simulink model "simu_rst_pendule"  (R2025b)
settings: Solver=ode45  StartTime=0.0  StopTime=30  MaxStep=0.01  RelTol=1e-3  EnableMultiTasking=on
undefined symbols (not defined in the file): g, H, l, R, S, sigbuilder_block, T
settings Model: Creator=2022-0702  LastModifiedBy=baki
settings SolverCC: AlgebraicLoopSolver=TrustRegion
settings DataIOCC: LimitDataPoints=on  SaveFormat=Array  SignalLoggingSaveFormat=ModelDataLogs  ReturnWorkspaceOutputs=off
settings OptimizationCC: InitFltsAndDblsToZero=on  LifeSpan=inf
settings DebuggingCC: SaveWithParameterizedLinksMsg=none  UnderspecifiedInitializationDetection=Classic  MergeDetectMultiDrivingBlocksExec=none  SignalResolutionControl=TryResolveAllWithWarning  SolverPrmCheckMsg=warning  MultiTaskDSMMsg=warning  MultiTaskCondExecSysMsg=none  FcnCallInpInsideContextMsg=warning  UnconnectedInputMsg=warning  UnconnectedOutputMsg=warning  UnconnectedLineMsg=warning  SFUnexpectedBacktrackingDiag=warning  SFNoUnconditionalDefaultTransitionDiag=warning  SFExecutionAtInitializationDiag=none  ArithmeticOperatorsInVariantConditions=warning
settings HardwareCC: ProdBitPerPointer=32.0  ProdBitPerSizeT=32.0  ProdBitPerPtrDiffT=32.0  ProdLargestAtomicFloat=None  ProdIntDivRoundTo=Undefined  ProdEndianess=Unspecified  ProdWordSize=32.0  ProdHWDeviceType=32-bit Generic
settings ModelReferenceCC: PropagateSignalLabelsOutOfModel=off
settings SFSimCC: SimUseLocalCustomCode=off  CustomCodeUndefinedFunction=UseInterfaceOnly
settings RTWCC: RTWUseLocalCustomCode=off  GPUComputeCapability=3.5
settings CodeAppCC: StateflowObjectComments=on
settings GRTTargetCC: TargetFcnLib=ansi_tfl_tmw.mat  TargetLangStandard=C89/C90 (ANSI)  CombineOutputUpdateFcns=off  GRTInterface=on
settings ConfigComp: CovMetricSettings=dw  CovSaveCumulativeToWorkspaceVar=on  CovSaveSingleToWorkspaceVar=on  CovExternalEMLEnable=off

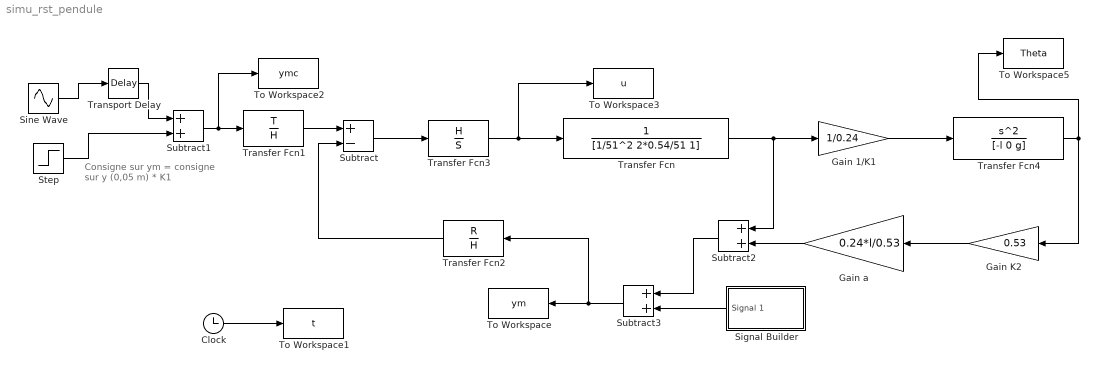
== system simu_rst_pendule ==
  note: Consigne sur ym
      | = consigne sur y
      | (0,05 m) * K1
  Clock : Clock
  Gain 1/K1 : Gain  Gain=1/0.24
  Gain K2 : Gain  Gain=0.53
  Gain a : Gain  Gain=0.24*l/0.53
  Signal Builder : Subsystem  Tag=STV Subsys  LoadFcn=sigbuilder_block('load');  StartFcn=sigbuilder_block('start');  StopFcn=sigbuilder_block('stop');  ClipboardFcn=sigbuilder_block('clipboard');  mask(Sigbuilder block){tuvar=[0:10]}
      mask help: Sigbuilder GUI
      mask init:
      | if ~strcmp(get_param(bdroot(gcbh),'SimulationStatus'),'stopped') tuvar = sigbuilder_block('maskInit'); end
      settings: CopyFcn=sigbuilder_block('copy');  DeleteFcn=sigbuilder_block('delete');  ModelCloseFcn=sigbuilder_block('modelClose');  PreSaveFcn=sigbuilder_block('preSave');  PauseFcn=sigbuilder_block('pause')  ContinueFcn=sigbuilder_block('continue')  NameChangeFcn=sigbuilder_block('namechange');  OpenFcn=sigbuilder_block('open',[203.25 117.75 671.25 404.25 ]);  CloseFcn=sigbuilder_block('close');
      mask Display: plot(0, 0, 100, 100,[2, 2, 32, 32, 2], [68, 8, 8, 68, 68],[32, 2], [38, 38], [32, 19, 2],[53, 60, 44], [32, 17, 17, 2],[16, 16, 31, 31]);txt = getActiveGroup(gcbh);text(2, 100, txt,'verticalAlignment', 'top');
  Sine Wave : Sin  SampleTime=0
  Step : Step  Time=15  SampleTime=0
  Subtract : Sum  Inputs=+-
  Subtract1 : Sum
  Subtract2 : Sum
  Subtract3 : Sum
  To Workspace : ToWorkspace  VariableName=ym  SampleTime=-1
  To Workspace1 : ToWorkspace  VariableName=t  SampleTime=-1
  To Workspace2 : ToWorkspace  VariableName=ymc  SampleTime=-1
  To Workspace3 : ToWorkspace  VariableName=u  SampleTime=-1
  To Workspace5 : ToWorkspace  VariableName=Theta  SampleTime=-1
  Transfer Fcn : TransferFcn  Numerator=1  Denominator=[1/51^2 2*0.54/51 1]
  Transfer Fcn1 : TransferFcn  Numerator=T  Denominator=H
  Transfer Fcn2 : TransferFcn  Numerator=R  Denominator=H
  Transfer Fcn3 : TransferFcn  Numerator=H  Denominator=S
  Transfer Fcn4 : TransferFcn  Numerator=[1 0 0]  Denominator=[-l 0 g]
  Transport Delay : TransportDelay  DelayTime=5  BufferSize=13312
  wires:
  Step/1 -> Subtract1/2
  Subtract1/1 -> To Workspace2/1, Transfer Fcn1/1
  Transfer Fcn1/1 -> Subtract/1
  Transfer Fcn2/1 -> Subtract/2
  Subtract/1 -> Transfer Fcn3/1
  Transfer Fcn3/1 -> Transfer Fcn/1, To Workspace3/1
  Transfer Fcn/1 -> Subtract2/1, Gain 1/K1/1
  Gain 1/K1/1 -> Transfer Fcn4/1
  Transfer Fcn4/1 -> To Workspace5/1, Gain K2/1
  Gain K2/1 -> Gain a/1
  Gain a/1 -> Subtract2/2
  Clock/1 -> To Workspace1/1
  Sine Wave/1 -> Transport Delay/1
  Transport Delay/1 -> Subtract1/1
  Subtract3/1 -> Transfer Fcn2/1, To Workspace/1
  Subtract2/1 -> Subtract3/1
  Signal Builder/1(Signal 1) -> Subtract3/2

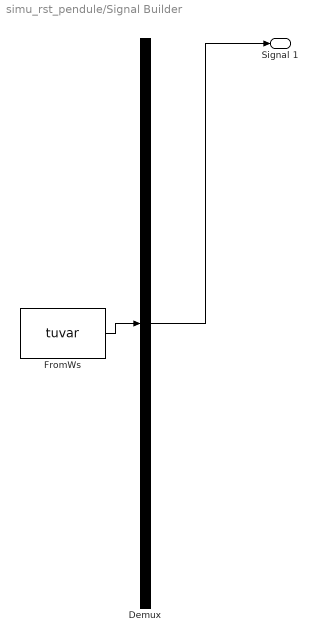
== system simu_rst_pendule/Signal Builder ==
  Demux : Demux  Tag=STV Demux  Outputs=1
      settings: DisplayOption=none
  FromWs : FromWorkspace  Tag=STV FromWs  VariableName=tuvar
  Signal 1 : Outport  Tag=STV Outport
  wires:
  Demux/1 -> Signal 1/1
  FromWs/1 -> Demux/1
